simulink model "AbstractFuelControl_M2_Navid"  (R2022b)
settings: Solver=ode23s  StartTime=0.0  StopTime=simTime  RelTol=1e-4  EnableMultiTasking=on
values from neighbouring files (symbols this model uses):
  c1 = 0.41328    [runMe.m]
  c10 = 1.0    (= 1)    [runMe.m]
  c11 = 14.7    [runMe.m]
  c12 = 0.9    [runMe.m]
  c13 = 0.04    [runMe.m]
  c14 = 0.14    [runMe.m]
  c2 = -0.366    [runMe.m]
  c23 = 1.0    (= 1)    [runMe.m]
  c24 = 1.0    (= 1)    [runMe.m]
  c25 = 1.0    (= 1)    [runMe.m]
  c3 = 0.08979    [runMe.m]
  c4 = -0.0337    [runMe.m]
  c5 = 0.0001    [runMe.m]
  c6 = 2.821    [runMe.m]
  c7 = -0.05231    [runMe.m]
  c8 = 0.10299    [runMe.m]
  c9 = -0.00063    [runMe.m]
  fault_time = 100    [runMe.m]
  i_init = 0    [runMe.m]
  p_est_init = 0.5455    [runMe.m]
  p_init = 0.725    [runMe.m]
settings Model: Creator=xjin  LastModifiedBy=jyoti
settings SolverCC: AlgebraicLoopSolver=TrustRegion
settings DataIOCC: ExternalInput=[simTime, en_speed]  SaveFormat=Array  SaveOutput=off  SaveTime=off  ReturnWorkspaceOutputs=off
settings OptimizationCC: LifeSpan=inf
settings DebuggingCC: AlgebraicLoopMsg=none  UnderspecifiedInitializationDetection=Classic  MergeDetectMultiDrivingBlocksExec=none  SolverPrmCheckMsg=warning  UnconnectedInputMsg=warning  UnconnectedOutputMsg=warning  UnconnectedLineMsg=warning  SFUnexpectedBacktrackingDiag=warning  SFNoUnconditionalDefaultTransitionDiag=warning  SFExecutionAtInitializationDiag=none  SFMachineParentedDataDiag=warning  ArithmeticOperatorsInVariantConditions=warning
settings HardwareCC: ProdBitPerPointer=32  ProdBitPerSizeT=32  ProdBitPerPtrDiffT=32  ProdLargestAtomicFloat=None  ProdIntDivRoundTo=Undefined  ProdEndianess=Unspecified  ProdWordSize=32  ProdHWDeviceType=32-bit Generic
settings ModelReferenceCC: PropagateSignalLabelsOutOfModel=off
settings SFSimCC: SimUseLocalCustomCode=off  CustomCodeUndefinedFunction=UseInterfaceOnly
settings RTWCC: RTWUseLocalCustomCode=off
settings CodeAppCC: StateflowObjectComments=on
settings GRTTargetCC: TargetLangStandard=C89/C90 (ANSI)
settings ConfigComp: CovMetricSettings=dw  CovSaveCumulativeToWorkspaceVar=on  CovSaveSingleToWorkspaceVar=on  CovExternalEMLEnable=off

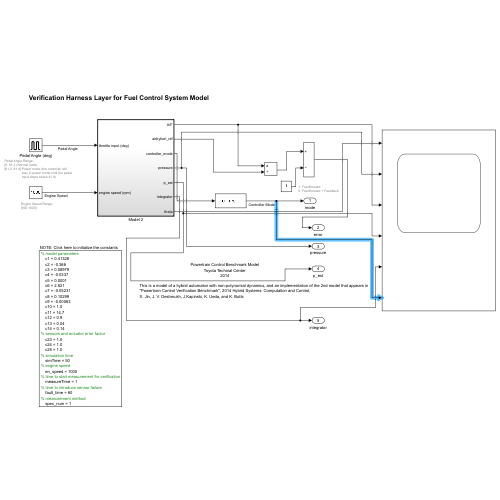
[thumbnail: Simulink's stored preview of the top-level diagram]
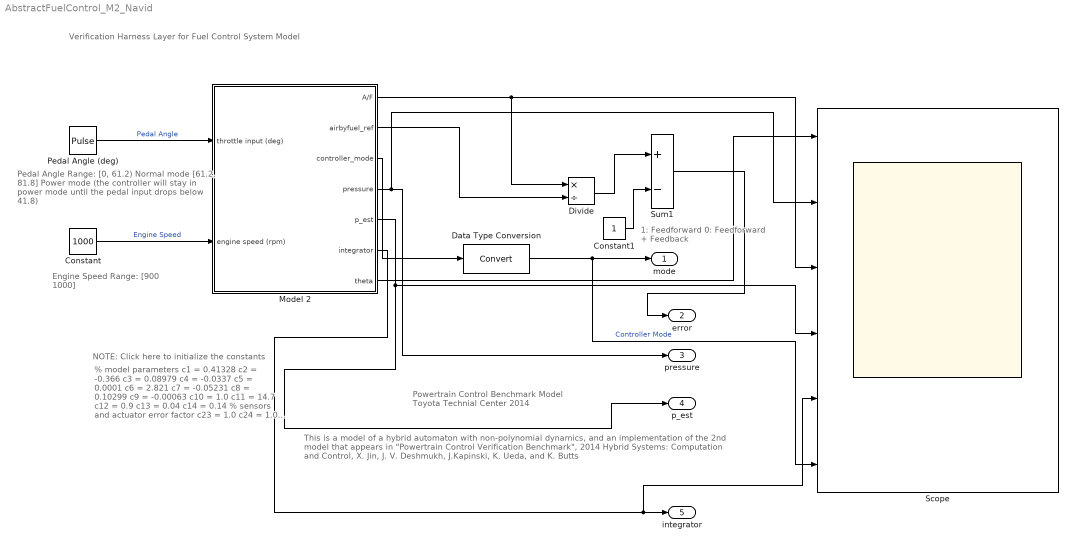
== system AbstractFuelControl_M2_Navid ==
  note: % model parameters
      |     c1 = 0.41328
      |     c2 = -0.366
      |     c3 = 0.08979
      |     c4 = -0.0337
      |     c5 = 0.0001
      |     c6 = 2.821
      |     c7 = -0.05231
      |     c8 = 0.10299
      |     c9 = -0.00063
      |     c10 = 1.0
      |     c11 = 14.7
      |     c12 = 0.9
      |     c13 = 0.04
      |     c14 = 0.14
      | % sensors and actuator error factor
      |     c23 = 1.0
      |     c24 = 1.0
      |     c25 = 1.0
      | % simulation time
      |     simTime = 50
      | % engine speed
      |     en_speed = 1000
      | % time to start measurement for verification
      |     measureTime = 1
      | % time to introduce sensor failure
      |     fault_time = 60
      | % measurement method
      |     spec_num = 1
  note: Verification Harness Layer for Fuel Control System Model
  note: Pedal Angle Range:
      | [0, 61.2) Normal mode
      | [61.2, 81.8] Power mode (the controller will
      |                    stay in power mode until the pedal
      |                    input drops below 41.8)
  note: Engine Speed Range:
      | [900 1000]
  note: 1: Feedforward
      | 0: Feedforward + Feedback
  note: This is a model of a hybrid automaton with non-polynomial dynamics, and an implementation of the 2nd model that appears in
      | "Powertrain Control Verification Benchmark", 2014 Hybrid Systems: Computation and Control,
      | X. Jin, J. V. Deshmukh, J.Kapinski, K. Ueda, and K. Butts
  note: Powertrain Control Benchmark Model
      | Toyota Technial Center
      | 2014
  note: NOTE: Click here to initialize the constants
  Constant : Constant  Value=1000
  Constant1 : Constant
  Data Type Conversion : DataTypeConversion  SaturateOnIntegerOverflow=off  RndMeth=Floor
  Divide : Product  Inputs=*/
  Model 2 : Subsystem  Priority=1  TreatAsAtomicUnit=on
  Pedal Angle (deg) : DiscretePulseGenerator  PulseType=Time based  Amplitude=50  Period=20  PulseWidth=50  PhaseDelay=3
  Scope : Scope  NumInputPorts=6
  Sum1 : Sum  Inputs=+-  InputSameDT=on  OutDataTypeStr=Inherit: Inherit via back propagation  RndMeth=Simplest
  mode : Outport
  error : Outport  Port=2
  pressure : Outport  Port=3
  p_est : Outport  Port=4
  integrator : Outport  Port=5
  wires:
  Constant/1 -> Model 2/2(engine speed (rpm))  "Engine Speed"
  Pedal Angle (deg)/1 -> Model 2/1(throttle input (deg))  "Pedal Angle"
  Data Type Conversion/1 -> Scope/6, mode/1  "Controller Mode"
  Model 2/2(airbyfuel_ref) -> Divide/2
  Sum1/1 -> error/1
  Model 2/1(A/F) -> Scope/3, Divide/1
  Constant1/1 -> Sum1/2
  Divide/1 -> Sum1/1
  Model 2/5(p_est) -> Scope/4, p_est/1
  Model 2/6(integrator) -> Scope/5, integrator/1
  Model 2/4(pressure) -> Scope/2, pressure/1
  Model 2/7(theta) -> Scope/1
  Model 2/3(controller_mode) -> Data Type Conversion/1

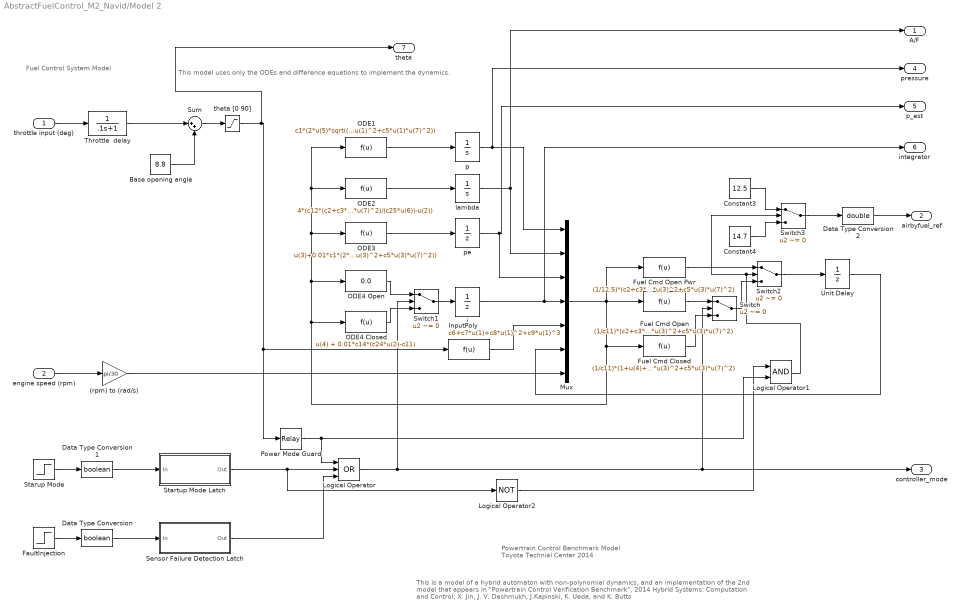
== system AbstractFuelControl_M2_Navid/Model 2 ==
  note: This model uses only the ODEs and difference equations to implement the dynamics.
  note: Fuel Control System Model
  note: This is a model of a hybrid automaton with non-polynomial dynamics, and an implementation of the 2nd model that appears in
      | "Powertrain Control Verification Benchmark", 2014 Hybrid Systems: Computation and Control,
      | X. Jin, J. V. Deshmukh, J.Kapinski, K. Ueda, and K. Butts
  note: Powertrain Control Benchmark Model
      | Toyota Technial Center
      | 2014
  throttle input (deg) : Inport  Description=[0, 81.2]
      settings: AttributesFormatString=%<Description>
  engine speed (rpm) : Inport  Description=[900,1100]  Port=2
      settings: AttributesFormatString=%<Description>
  (rpm) to (rad/s) : Gain  Gain=pi/30
  Base opening angle : Constant  Value=8.8
  Constant3 : Constant  Value=12.5
  Constant4 : Constant  Value=14.7
  Data Type Conversion : DataTypeConversion  OutDataTypeStr=boolean  SaturateOnIntegerOverflow=off  RndMeth=Floor
  Data Type Conversion1 : DataTypeConversion  OutDataTypeStr=boolean  SaturateOnIntegerOverflow=off  RndMeth=Floor
  Data Type Conversion2 : DataTypeConversion  OutDataTypeStr=double  SaturateOnIntegerOverflow=off  RndMeth=Floor
  FaultInjection : Step  Time=fault_time  SampleTime=0
      settings: AttributesFormatString=1: Failure\n0: Normal
  Fuel Cmd Closed : Fcn  Expr=(1/c11)*(1+u(4)+c13*(c24*u(2)-c11))*(c2+c3*u(7)*u(3)+c4*u(7)*u(3)^2+c5*u(3)*u(7)^2)
  Fuel Cmd Open : Fcn  Expr=(1/c11)*(c2+c3*u(7)*u(3)+c4*u(7)*u(3)^2+c5*u(3)*u(7)^2)
  Fuel Cmd Open Pwr : Fcn  Expr=(1/12.5)*(c2+c3*u(7)*u(3)+c4*u(7)*u(3)^2+c5*u(3)*u(7)^2)
  InputPoly : Fcn  Expr=c6+c7*u(1)+c8*u(1)^2+c9*u(1)^3
  Logical Operator : Logic  Operator=OR  Inputs=3  AllPortsSameDT=off  OutDataTypeStr=boolean
  Logical Operator1 : Logic  AllPortsSameDT=off  OutDataTypeStr=boolean
  Logical Operator2 : Logic  Operator=NOT  Inputs=3  AllPortsSameDT=off  OutDataTypeStr=boolean
  Mux : Mux  Inputs=7
  ODE1 : Fcn  Expr=c1*(2*u(5)*sqrt((u(1)/c10)-(u(1)/c10)^2) - c12*(c2+c3*u(7)*u(1)+c4*u(7)*u(1)^2+c5*u(1)*u(7)^2))
  ODE2 : Fcn  Expr=4*(c12*(c2+c3*u(7)*u(1)+c4*u(7)*u(1)^2+c5*u(1)*u(7)^2)/(c25*u(6))-u(2))
  ODE3 : Fcn  Expr=u(3)+0.01*c1*(2*c23*u(5)*sqrt((u(1)/c10)-(u(1)/c10)^2) - (c2+c3*u(7)*u(3)+c4*u(7)*u(3)^2+c5*u(3)*u(7)^2))
  ODE4 Closed : Fcn  Expr=u(4) + 0.01*c14*(c24*u(2)-c11)
  ODE4 Open : Fcn  Expr=0.0
  Power Mode Guard : Relay  OnSwitchValue=70  OffSwitchValue=50  SampleTime=0.01
  Sensor Failure Detection Latch : Subsystem  TreatAsAtomicUnit=on
  Startup Mode Latch : Subsystem  TreatAsAtomicUnit=on
  Starup Mode : Step  Time=10  Before=1  After=0  SampleTime=0
  Sum : Sum  Inputs=|++
  Switch{,1..3} (4 alike) : Switch  Criteria=u2 ~= 0  SaturateOnIntegerOverflow=off  InputSameDT=off
  Throttle  delay : TransferFcn  Denominator=[.1 1]
  Unit Delay : UnitDelay  InitialCondition=0.6537  SampleTime=0.01  HasFrameUpgradeWarning=on
  i : UnitDelay  InitialCondition=i_init  SampleTime=0.01  HasFrameUpgradeWarning=on
  lambda : Integrator  InitialCondition=14.7
  p : Integrator  InitialCondition=p_init
  pe : UnitDelay  InitialCondition=p_est_init  SampleTime=0.01  HasFrameUpgradeWarning=on
  theta [0 90] : Saturate  UpperLimit=90  LowerLimit=0
  A/F : Outport
  airbyfuel_ref : Outport  Port=2
  controller_mode : Outport  Port=3
  pressure : Outport  Port=4
  p_est : Outport  Port=5
  integrator : Outport  Port=6
  theta : Outport  Port=7
  wires:
  theta [0 90]/1 -> theta/1, Power Mode Guard/1, InputPoly/1
  Base opening angle/1 -> Sum/2
  ODE1/1 -> p/1
  Mux/1 -> Fuel Cmd Closed/1, ODE1/1, ODE2/1, ODE3/1, ODE4 Open/1, ODE4 Closed/1, Fuel Cmd Open/1, Fuel Cmd Open Pwr/1
  InputPoly/1 -> Mux/5
  Sum/1 -> theta [0 90]/1
  ODE3/1 -> pe/1
  ODE2/1 -> lambda/1
  p/1 -> pressure/1, Mux/1
  pe/1 -> p_est/1, Mux/3
  i/1 -> integrator/1, Mux/4
  throttle input (deg)/1 -> Throttle  delay/1
  lambda/1 -> Mux/2, A/F/1
  Fuel Cmd Open/1 -> Switch/1
  Fuel Cmd Closed/1 -> Switch/3
  Switch1/1 -> i/1
  ODE4 Open/1 -> Switch1/1
  ODE4 Closed/1 -> Switch1/3
  Switch/1 -> Switch2/3
  Unit Delay/1 -> Mux/6
  FaultInjection/1 -> Data Type Conversion/1
  Data Type Conversion/1 -> Sensor Failure Detection Latch/1(In)
  Logical Operator/1 -> Switch1/2, Switch/2, controller_mode/1
  Sensor Failure Detection Latch/1(Out) -> Logical Operator/3
  Startup Mode Latch/1(Out) -> Logical Operator2/1, Logical Operator/2
  Starup Mode/1 -> Data Type Conversion1/1
  Data Type Conversion1/1 -> Startup Mode Latch/1(In)
  Switch2/1 -> Unit Delay/1
  Fuel Cmd Open Pwr/1 -> Switch2/1
  engine speed (rpm)/1 -> (rpm) to (rad/s)/1
  (rpm) to (rad/s)/1 -> Mux/7
  Switch3/1 -> Data Type Conversion2/1
  Constant3/1 -> Switch3/1
  Constant4/1 -> Switch3/3
  Power Mode Guard/1 -> Logical Operator/1, Logical Operator1/2
  Data Type Conversion2/1 -> airbyfuel_ref/1
  Logical Operator2/1 -> Logical Operator1/1
  Logical Operator1/1 -> Switch3/2, Switch2/2
  Throttle  delay/1 -> Sum/1

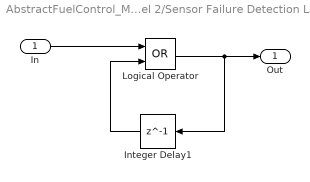
== system AbstractFuelControl_M2_Navid/Model 2/Sensor Failure Detection Latch ==
  In : Inport
  Integer Delay1 : Delay  DelayLength=1  SampleTime=0.01
  Logical Operator : Logic  Operator=OR  AllPortsSameDT=off
  Out : Outport
  wires:
  Logical Operator/1 -> Out/1, Integer Delay1/1
  Integer Delay1/1 -> Logical Operator/2
  In/1 -> Logical Operator/1

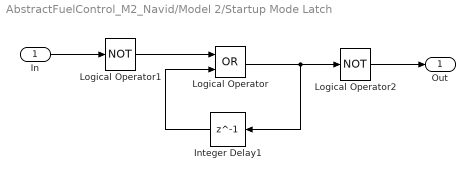
== system AbstractFuelControl_M2_Navid/Model 2/Startup Mode Latch ==
  In : Inport
  Integer Delay1 : Delay  DelayLength=1  SampleTime=0.01
  Logical Operator : Logic  Operator=OR  AllPortsSameDT=off
  Logical Operator1 : Logic  Operator=NOT  AllPortsSameDT=off
  Logical Operator2 : Logic  Operator=NOT  AllPortsSameDT=off
  Out : Outport
  wires:
  In/1 -> Logical Operator1/1
  Integer Delay1/1 -> Logical Operator/2
  Logical Operator/1 -> Integer Delay1/1, Logical Operator2/1
  Logical Operator1/1 -> Logical Operator/1
  Logical Operator2/1 -> Out/1
